simulink model "a3"  (R2020a)
settings: Solver=VariableStepAuto  StartTime=0.0  StopTime=2  RelTol=1e-3
undefined symbols (not defined in the file): sigbuilder_block
settings Model: Creator=bill2  LastModifiedBy=bill2
settings DataIOCC: Refine=10

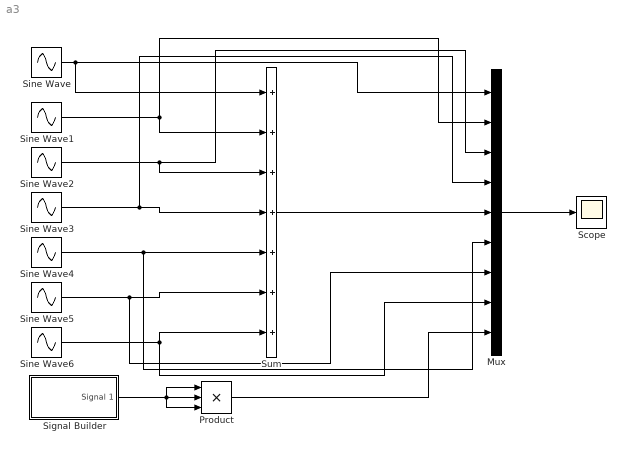
== system a3 ==
  Mux : Mux  Inputs=9
  Product : Product  Inputs=3
  Scope : Scope
  Signal Builder : Subsystem  Tag=STV Subsys  LoadFcn=sigbuilder_block('load');  StartFcn=sigbuilder_block('start');  StopFcn=sigbuilder_block('stop');  ClipboardFcn=sigbuilder_block('clipboard');  mask(Sigbuilder block){tuvar=[0:10]}
      mask help: Simulink:masks:SigbuilderBlock_MD
      mask init:
      | if ~strcmp(get_param(bdroot(gcbh),'SimulationStatus'),'stopped') tuvar = sigbuilder_block('maskInit'); end
      settings: CopyFcn=sigbuilder_block('copy');  DeleteFcn=sigbuilder_block('delete');  ModelCloseFcn=sigbuilder_block('modelClose');  PreSaveFcn=sigbuilder_block('preSave');  PauseFcn=sigbuilder_block('pause');  ContinueFcn=sigbuilder_block('continue');  NameChangeFcn=sigbuilder_block('namechange');  OpenFcn=sigbuilder_block('open',[1440 -162 1440 753.6 ]);  CloseFcn=sigbuilder_block('close');
      mask Display: plot(0, 0, 100, 100,[2, 2, 32, 32, 2], [68, 8, 8, 68, 68],[32, 2], [38, 38], [32, 19, 2],[53, 60, 44], [32, 17, 17, 2],[16, 16, 31, 31]);txt = getActiveGroup(gcbh);text(2, 100, txt,'verticalAlignment', 'top');
  Sine Wave : Sin  Amplitude=2*(pi^2-6)  Frequency=2*pi  SampleTime=0
  Sine Wave1 : Sin  Amplitude=-(1/4)*(pi^2*4-6)  Frequency=4*pi  SampleTime=0
  Sine Wave2 : Sin  Amplitude=(2/27)*(pi^2*9-6)  Frequency=6*pi  SampleTime=0
  Sine Wave3 : Sin  Amplitude=-(1/32)*(pi^2*16-6)  Frequency=8*pi  SampleTime=0
  Sine Wave4 : Sin  Amplitude=(2/125)*(pi^2*25-6)  Frequency=10*pi  SampleTime=0
  Sine Wave5 : Sin  Amplitude=-(1/108)*(pi^2*36-6)  Frequency=12*pi  SampleTime=0
  Sine Wave6 : Sin  Amplitude=(2/343)*(pi^2*49-6)  Frequency=14*pi  SampleTime=0
  Sum : Sum  Inputs=7
  wires:
  Signal Builder/1(Signal 1) -> Product/3, Product/1, Product/2
  Sine Wave1/1 -> Mux/2, Sum/2
  Sine Wave2/1 -> Mux/3, Sum/3
  Sine Wave3/1 -> Mux/4, Sum/4
  Sine Wave4/1 -> Mux/6, Sum/5
  Sine Wave5/1 -> Mux/7, Sum/6
  Sine Wave6/1 -> Mux/8, Sum/7
  Sum/1 -> Mux/5
  Mux/1 -> Scope/1
  Sine Wave/1 -> Sum/1, Mux/1
  Product/1 -> Mux/9

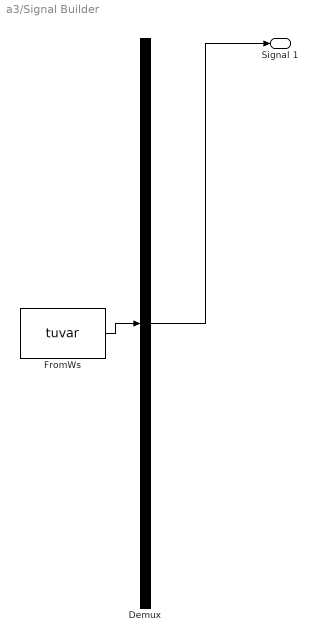
== system a3/Signal Builder ==
  Demux : Demux  Tag=STV Demux  Outputs=1
      settings: DisplayOption=none
  FromWs : FromWorkspace  Tag=STV FromWs  VariableName=tuvar
      SigBuilderData=|
      | common.afterFinalStr = 'Extrapolate'
      | common.sampleTime = 0
      | dataSet.timeRange = [0 2]
      | dataSet.name = 'Group 1'
      | sbobj.Groups.Name = 'Group 1'
      | sbobj.Groups.Signals.Name = 'Signal 1'
      | sbobj.Groups.Signals.XData = [0 0.5 0.5 1 1.5 1.5 2]
      | sbobj.Groups.Signals.YData = [0 3.14159265359 -3.14159265359 0 3.14159265359 -3.14159265359 0]
      | sbobj.Groups.TimeRange = [0 2]
  Signal 1 : Outport  Tag=STV Outport
  wires:
  Demux/1 -> Signal 1/1
  FromWs/1 -> Demux/1
